simulink model "PCellVoltageDerate"  (R2024b)
settings: Solver=FixedStepAuto  StartTime=0.0  StopTime=10.0  RelTol=1e-3  EnableMultiTasking=on
settings Model: DataDictionary=Master_Dictionary.sldd  EnableAccessToBaseWorkspace=off  Creator=torni  LastModifiedBy=Will
settings OptimizationCC: DefaultParameterBehavior=Inlined  EnhancedBackFolding=on  PassReuseOutputArgsAs=Individual arguments  ZeroExternalMemoryAtStartup=off  ZeroInternalMemoryAtStartup=off  MaxStackSize=8192  OptimizeBlockOrder=speed  DifferentSizesBufferReuse=on  OptimizationCustomize=off  EfficientTunableParamExpr=on
settings DebuggingCC: ParameterTunabilityLossMsg=error
settings HardwareCC: ProdBitPerPointer=32  ProdBitPerSizeT=32  ProdBitPerPtrDiffT=32  ProdLargestAtomicInteger=Long  ProdLargestAtomicFloat=Double  ProdWordSize=32  ProdLongLongMode=on  ProdHWDeviceType=ARM Compatible->ARM Cortex-M
settings SFSimCC: MATLABDynamicMemAlloc=off
settings RTWCC: Description=Embedded Coder  SystemTargetFile=ert.tlc  HardwareBoard=STM32H7xx Based (Single-core)  TemplateMakefile=ert_default_tmf  Toolchain=GNU Tools for ARM Embedded Processors
settings CodeAppCC: ForceParamTrailComments=on  IgnoreCustomStorageClasses=off  OperatorAnnotations=on  SimulinkDataObjDesc=on  SFDataObjDesc=on  InsertBlockDesc=on
settings ERTTargetCC: TargetLangStandard=C99 (ISO)  CodeReplacementLibrary=ARM Cortex-M  ExtModeTransport=3  ExtModeStaticAlloc=on  ExtModeStaticAllocSize=2048  ExtModeMexFile=ext_xcp  ExtModeIntrfLevel=Level2 - Open

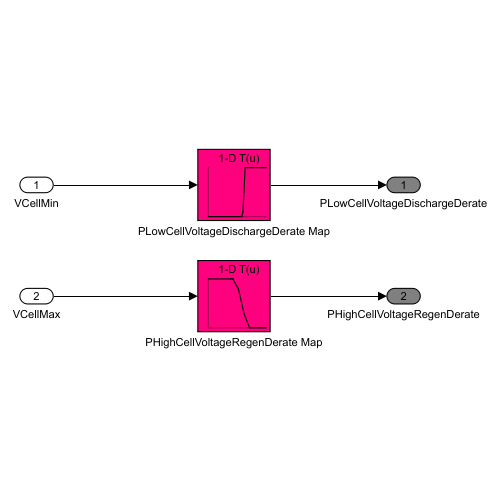
[thumbnail: Simulink's stored preview of the top-level diagram]
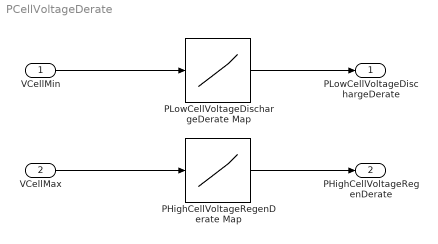
== system PCellVoltageDerate ==
  "VCellMin " : Inport  OutDataTypeStr=double
  VCellMax : Inport  Port=2  OutDataTypeStr=double
  PHighCellVoltageRegenDerate Map : Lookup_n-D  NumberOfTableDimensions=1  BreakpointsForDimension1=[2.9,3.7,3.8,4,4.2,4.4,5]  Table=[100,100,100,80,30,0,0]  InternalRulePriority=Speed  RndMeth=Simplest
  PLowCellVoltageDischargeDerate Map : Lookup_n-D  NumberOfTableDimensions=1  BreakpointsForDimension1=[0,2.9,3,3.1,3.2,5]  Table=[0,0,7.8,39,78,78]  InternalRulePriority=Speed  RndMeth=Simplest
  PLowCellVoltageDischargeDerate : Outport  OutDataTypeStr=double  VectorParamsAs1DForOutWhenUnconnected=off
  PHighCellVoltageRegenDerate : Outport  Port=2  OutDataTypeStr=double  VectorParamsAs1DForOutWhenUnconnected=off
  wires:
  "VCellMin "/1 -> PLowCellVoltageDischargeDerate Map/1
  PLowCellVoltageDischargeDerate Map/1 -> PLowCellVoltageDischargeDerate/1
  VCellMax/1 -> PHighCellVoltageRegenDerate Map/1
  PHighCellVoltageRegenDerate Map/1 -> PHighCellVoltageRegenDerate/1
